simulink model "mdl_filterung"  (Simulink 10.2)
settings: Solver=FixedStepDiscrete  StartTime=0.0  StopTime=t_end  FixedStep=t_sample  RelTol=1e-3  EnableMultiTasking=on
PostLoadFcn:
  | , if any(exist('dsrtsu_mdlpostloadfcn', 'file') == [2, 3, 6]), try dsrtsu_mdlpostloadfcn('Execute', bdroot); catch fprintf('Error in PostLoadFcn (dsrtsu_mdlpostloadfcn) for model "%s":\n %s\n', bdroot, lasterr); end, end,
values from neighbouring files (symbols this model uses):
  a = [1 -3.18063854887 3.86119434899 -2.11215535511 0.438265142262]    [data_iir.mat]
  b = [0.000416599204407 0.00166639681763 0.00249959522644 0.00166639681763 0.000416599204407]    [data_iir.mat]
  t_sample = 0.001    [data_iir.mat]    (also in generate_test_data.m)
settings Model: DSRTSU_INTERNAL_RTI_VER=360  DSRTSU_INTERNAL_RTI_TYPE=rti1103  Creator=Schaper  LastModifiedBy=werne
settings DataIOCC: LimitDataPoints=on
settings OptimizationCC: BlockReduction=off  OptimizeBlockIOStorage=off  BufferReuse=off  GlobalBufferReuse=off  ExpressionFolding=off  ExpressionDepthLimit=2147483647  LocalBlockOutputs=off
settings DebuggingCC: SolverPrmCheckMsg=warning  AllowSymbolicDim=off  StateNameClashWarn=warning
settings HardwareCC: ProdIntDivRoundTo=Zero  ProdEndianess=BigEndian  ProdHWDeviceType=Generic->Custom  TargetIntDivRoundTo=Zero  TargetEndianess=BigEndian  TargetHWDeviceType=Generic->Custom
settings RTWCC: Description=dSPACE DS1103 Hardware Platform  SystemTargetFile=rti1103.tlc  MakeCommand=make_rti  TemplateMakefile=rti1103.tmf
settings STFCustomTargetCC: ParMdlRefBuildCompliant=on  MatFileLogging=on  CPPClassGenCompliant=on  SystemTargetFile=rti1103.tlc
settings GRTTargetCC: CompOptLevelCompliant=off  ConcurrentExecutionCompliant=off  UseToolchainInfoCompliant=off  ExtModeMexFile=noextcomm
settings CustomProperty: DataType=RTWOptions_EnumType_C__Programme_dSPACE66_matlab_rti1103_tlc_rti1103_1InitialSimState  Value=RUN
settings EnumStrPairs: String=RUN

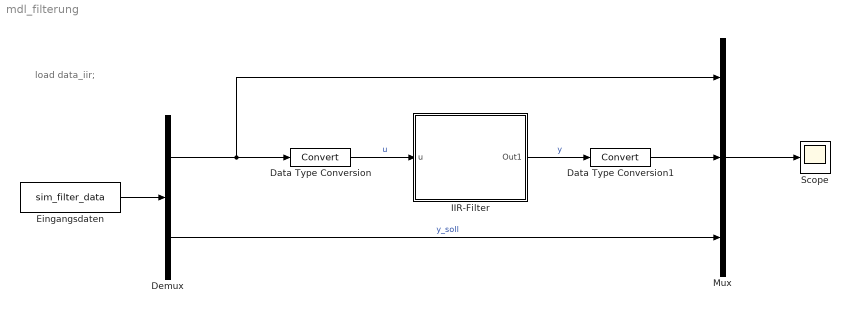
== system mdl_filterung ==
  note: load data_iir;
  Data Type Conversion : DataTypeConversion
  Data Type Conversion1 : DataTypeConversion
  Demux : Demux  Outputs=2
  Eingangsdaten : FromWorkspace  VariableName=sim_filter_data  SampleTime=t_sample
  IIR-Filter : Subsystem  mask{b=b, a=a}
      mask prompts: b "Zähler-Koeffizienten b"; a "Nenner-Koeffizienten a"
  Mux : Mux  Inputs=3
  Scope : Scope
  wires:
  Mux/1 -> Scope/1
  Data Type Conversion/1 -> IIR-Filter/1(u)  "u"
  IIR-Filter/1(Out1) -> Data Type Conversion1/1  "y"
  Eingangsdaten/1 -> Demux/1
  Demux/1 -> Mux/1, Data Type Conversion/1
  Demux/2 -> Mux/3  "y_soll"
  Data Type Conversion1/1 -> Mux/2

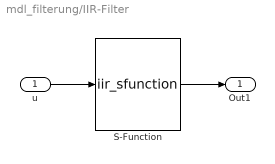
== system mdl_filterung/IIR-Filter ==
  u : Inport
  S-Function : S-Function  FunctionName=iir_sfunction  Parameters=a,b  SFunctionDeploymentMode=off  EnableBusSupport=off
  Out1 : Outport
  wires:
  u/1 -> S-Function/1
  S-Function/1 -> Out1/1
